simulink model "test_d_v_p"  (Simulink 6.2)
settings: Solver=ode45  StartTime=0.0  StopTime=30000  RelTol=1e-3
undefined symbols (not defined in the file or in its folder): ant_bits, blockCountBits, blockRowBits
libraries: xbsIndex_r3 x843, xps_library x50, casper_library x17
(part 1 of 6)
settings Model: LastModifiedBy=Jason Manley
settings DebuggingCC: SolverPrmCheckMsg=warning

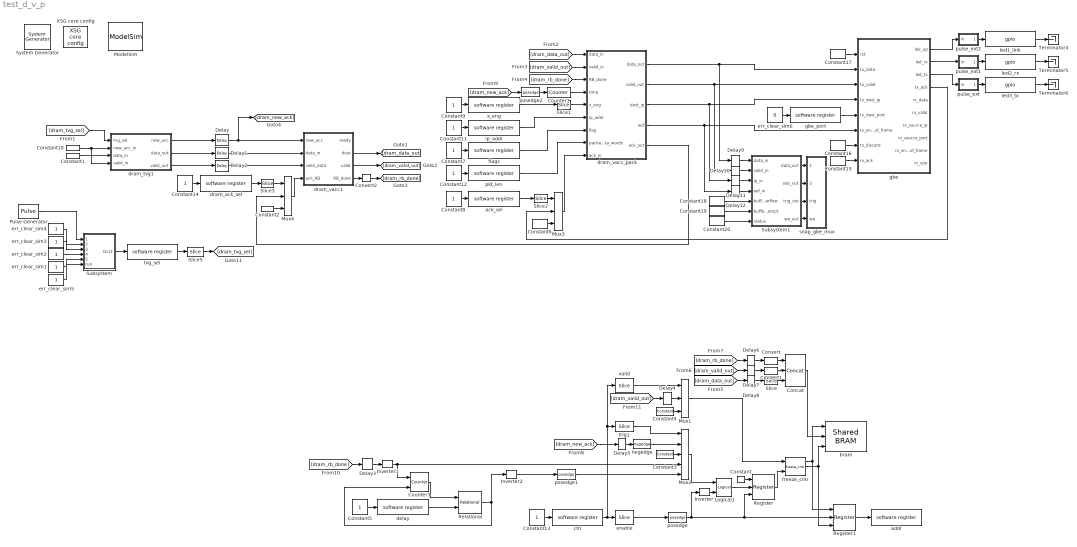
== system test_d_v_p ==
  " System Generator" : xbsIndex_r3/ System Generator  Tag=genX  xilinxfamily=Virtex2P  part=xc2vp70  speed=-7  package=ff1704  synthesis_tool=XST  directory=./test_d_v_p/sysgen  testbench=off  simulink_period=1  sysclk_period=4.878  incr_netlist=off  trim_vbits=Everywhere in SubSystem  dbl_ovrd=According to Block Masks  core_generation=According to Block Masks  run_coregen=off  deprecated_control=off  eval_field=0
      settings: AttributesFormatString=System\nGenerator
  Concat : xbsIndex_r3/Concat  num_inputs=3  explicit_period=off  period=1  dbl_ovrd=off
  Constant{,2..4} (4 alike) : xbsIndex_r3/Constant  const=1  equ=P=C  arith_type=Boolean  n_bits=1  bin_pt=0  opselect=C  inp2=PCIN>>17  opr=+  inp1=P  carry=CIN  iostate=0  explicit_period=on  period=1  dbl_ovrd=off
  Constant1 : xbsIndex_r3/Constant  const=0  equ=P=C  arith_type=Unsigned  n_bits=128  bin_pt=0  opselect=C  inp2=PCIN>>17  opr=+  inp1=P  carry=CIN  iostate=0  explicit_period=on  period=1  dbl_ovrd=off
  Constant10 : xbsIndex_r3/Constant  const=0  equ=P=C  arith_type=Boolean  n_bits=1  bin_pt=0  opselect=C  inp2=PCIN>>17  opr=+  inp1=P  carry=CIN  iostate=0  explicit_period=on  period=1  dbl_ovrd=off
  Constant{5,7..9,11..14} (8 alike) : Constant
  Constant15 : xbsIndex_r3/Constant  const=1  equ=P=C  arith_type=Boolean  n_bits=32  bin_pt=0  opselect=C  inp2=PCIN>>17  opr=+  inp1=P  carry=CIN  iostate=0  explicit_period=on  period=1  dbl_ovrd=off
  Constant{16..19} (4 alike) : xbsIndex_r3/Constant  const=0  equ=P=C  arith_type=Boolean  n_bits=32  bin_pt=0  opselect=C  inp2=PCIN>>17  opr=+  inp1=P  carry=CIN  iostate=0  explicit_period=on  period=1  dbl_ovrd=off
  Constant20 : xbsIndex_r3/Constant  const=0  equ=P=C  arith_type=Unsigned  n_bits=9  bin_pt=0  opselect=C  inp2=PCIN>>17  opr=+  inp1=P  carry=CIN  iostate=0  explicit_period=on  period=1  dbl_ovrd=off
  Constant6 : xbsIndex_r3/Constant  const=1  equ=P=C  arith_type=Boolean  n_bits=32  bin_pt=0  opselect=C  inp2=PCIN>>17  opr=+  inp1=P  carry=CIN  iostate=0  explicit_period=on  period=1  dbl_ovrd=off
  Convert : xbsIndex_r3/Convert  arith_type=Unsigned  n_bits=1  bin_pt=0  quantization=Truncate  overflow=Wrap  latency=0  explicit_period=off  period=1  dbl_ovrd=off  show_param=off  inserted_by_tool=off  pipeline=off
      settings: xl_area=[0, 0, 0, 0, 0, 0, 0]
  Convert1 : xbsIndex_r3/Convert  arith_type=Unsigned  n_bits=1  bin_pt=0  quantization=Truncate  overflow=Wrap  latency=0  explicit_period=off  period=1  dbl_ovrd=off  show_param=off  inserted_by_tool=off  pipeline=off
      settings: xl_area=[0, 0, 0, 0, 0, 0, 0]
  Convert2 : xbsIndex_r3/Convert  arith_type=Boolean  n_bits=1  bin_pt=0  quantization=Truncate  overflow=Wrap  latency=0  explicit_period=off  period=1  dbl_ovrd=off  show_param=off  inserted_by_tool=off  pipeline=off
      settings: xl_area=[0, 0, 0, 0, 0, 0, 0]
  Counter1 : xbsIndex_r3/Counter  cnt_type=Free Running  n_bits=64  bin_pt=0  arith_type=Unsigned  start_count=0  cnt_to=1023  cnt_by_val=1  operation=Up  explicit_period=on  period=1  load_pin=off  rst=off  en=on  dbl_ovrd=off  show_param=off  use_rpm=on  gen_core=off
      settings: xl_area=[0, 0, 0, 0, 0, 0, 0]
  Counter3 : xbsIndex_r3/Counter  cnt_type=Free Running  n_bits=32  bin_pt=0  arith_type=Unsigned  start_count=0  cnt_to=1023  cnt_by_val=1  operation=Up  explicit_period=on  period=1  load_pin=off  rst=on  en=on  dbl_ovrd=off  show_param=off  use_rpm=on  gen_core=off
      settings: xl_area=[0, 0, 0, 0, 0, 0, 0]
  Delay{,1..12} (13 alike) : xbsIndex_r3/Delay  latency=5  reg_retiming=on  explicit_period=off  period=1  en=off  accept_only_valid=off  init_zero=on  dbl_ovrd=off  show_param=off
      settings: xl_area=[0, 0, 0, 0, 0, 0, 0]
  Inverter : xbsIndex_r3/Inverter  latency=0  explicit_period=off  period=1  en=off  dbl_ovrd=off  show_param=off
      settings: xl_area=[0, 0, 0, 0, 0, 0, 0]
  Inverter1 : xbsIndex_r3/Inverter  latency=0  explicit_period=off  period=1  en=off  dbl_ovrd=off  show_param=off
      settings: xl_area=[0, 0, 0, 0, 0, 0, 0]
  Inverter2 : xbsIndex_r3/Inverter  latency=0  explicit_period=off  period=1  en=off  dbl_ovrd=off  show_param=off
      settings: xl_area=[0, 0, 0, 0, 0, 0, 0]
  Logical1 : xbsIndex_r3/Logical  logical_function=AND  inputs=2  precision=Full  arith_type=Unsigned  n_bits=8  bin_pt=2  align_bp=on  latency=0  explicit_period=off  period=1  en=off  dbl_ovrd=off  show_param=off
      settings: xl_area=[0, 0, 0, 0, 0, 0, 0]
  ModelSim : xbsIndex_r3/ModelSim  dir=./modelsim  waveform=on  leave_open=on  skip_compile=off  custom_scripts=off  startup_timeout=40
  Mux1 : xbsIndex_r3/Mux  inputs=2  precision=Full  arith_type="Signed  (2's comp)"  n_bits=8  bin_pt=2  quantization=Truncate  overflow=Wrap  latency=0  explicit_period=off  period=1  en=off  dbl_ovrd=off  show_param=off  mux_type=off  use_rpm=off  gen_core=off
      settings: xl_area=[0, 0, 0, 0, 0, 0, 0]
  Mux2 : xbsIndex_r3/Mux  inputs=4  precision=Full  arith_type="Signed  (2's comp)"  n_bits=8  bin_pt=2  quantization=Truncate  overflow=Wrap  latency=0  explicit_period=off  period=1  en=off  dbl_ovrd=off  show_param=off  mux_type=off  use_rpm=off  gen_core=off
      settings: xl_area=[0, 0, 0, 0, 0, 0, 0]
  Mux3 : xbsIndex_r3/Mux  inputs=2  precision=Full  arith_type="Signed  (2's comp)"  n_bits=8  bin_pt=2  quantization=Truncate  overflow=Wrap  latency=0  explicit_period=off  period=1  en=off  dbl_ovrd=off  show_param=off  mux_type=off  use_rpm=off  gen_core=off
      settings: xl_area=[0, 0, 0, 0, 0, 0, 0]
  Mux4 : xbsIndex_r3/Mux  inputs=2  precision=Full  arith_type="Signed  (2's comp)"  n_bits=8  bin_pt=2  quantization=Truncate  overflow=Wrap  latency=0  explicit_period=off  period=1  en=off  dbl_ovrd=off  show_param=off  mux_type=off  use_rpm=off  gen_core=off
      settings: xl_area=[0, 0, 0, 0, 0, 0, 0]
  Pulse Generator : DiscretePulseGenerator  Period=3000  PhaseDelay=600
  Register : xbsIndex_r3/Register  init=0  reg_only_valid=off  explicit_period=off  period=1  rst=on  en=on  out_en=off  dbl_ovrd=off  show_param=off
      settings: xl_area=[0, 0, 0, 0, 0, 0, 0]
  Register1 : xbsIndex_r3/Register  init=0  reg_only_valid=off  explicit_period=off  period=1  rst=on  en=on  out_en=off  dbl_ovrd=off  show_param=off
      settings: xl_area=[0, 0, 0, 0, 0, 0, 0]
  Relational : xbsIndex_r3/Relational  mode=a<=b  latency=0  explicit_period=off  period=1  en=off  dbl_ovrd=off  show_param=off
      settings: xl_area=[0, 0, 0, 0, 0, 0, 0]
  Slice : xbsIndex_r3/Slice  mode=Lower Bit Location + Width  nbits=30  bit1=0  base1=MSB of Input  bit0=0  base0=LSB of Input  boolean_output=off  explicit_period=off  period=1  dbl_ovrd=off
  Slice1 : xbsIndex_r3/Slice  mode=Lower Bit Location + Width  nbits=16  bit1=0  base1=MSB of Input  bit0=0  base0=LSB of Input  boolean_output=off  explicit_period=off  period=1  dbl_ovrd=off
  Slice2 : xbsIndex_r3/Slice  mode=Lower Bit Location + Width  nbits=1  bit1=0  base1=MSB of Input  bit0=0  base0=LSB of Input  boolean_output=off  explicit_period=off  period=1  dbl_ovrd=off
  Slice3 : xbsIndex_r3/Slice  mode=Lower Bit Location + Width  nbits=1  bit1=0  base1=MSB of Input  bit0=0  base0=LSB of Input  boolean_output=off  explicit_period=off  period=1  dbl_ovrd=off
  Slice5 : xbsIndex_r3/Slice  mode=Lower Bit Location + Width  nbits=6  bit1=0  base1=MSB of Input  bit0=9  base0=LSB of Input  boolean_output=off  explicit_period=off  period=1  dbl_ovrd=off
  Subsystem : Subsystem
  Subsystem1 : Subsystem
  Terminator4 : Terminator
  Terminator5 : Terminator
  Terminator6 : Terminator
  XSG core config : xps_library/XSG core config  Tag=xps:xsg  hw_sys=BEE2_usr  ibob_linux=off  clk_src=sys_clk2x  gpio_clk_io_group=iBOB:sma  gpio_clk_bit_index=0  clk_rate=205  sample_period=1  synthesis_tool=XST  mpc_type=powerpc405
  ack_sel : xps_library/software register  Tag=xps:sw_reg  io_dir=From Processor  arith_type=Unsigned  bitwidth=32  bin_pt=0  sample_period=1  gw_name=test_d_v_p_ack_sel_user_data_out
  addr : xps_library/software register  Tag=xps:sw_reg  io_dir=To Processor  arith_type=Unsigned  bitwidth=32  bin_pt=0  sample_period=1  gw_name=test_d_v_p_addr_user_data_in
  bram : xps_library/Shared BRAM  Tag=xps:bram  arith_type=Unsigned  addr_width=14  data_width=32  data_bin_pt=0  init_vals=0  sample_rate=1
  ctrl : xps_library/software register  Tag=xps:sw_reg  io_dir=From Processor  arith_type=Unsigned  bitwidth=32  bin_pt=0  sample_period=1  gw_name=test_d_v_p_ctrl_user_data_out
  delay : xps_library/software register  Tag=xps:sw_reg  io_dir=From Processor  arith_type=Unsigned  bitwidth=32  bin_pt=0  sample_period=1  gw_name=test_d_v_p_delay_user_data_out
  dram_ack_sel : xps_library/software register  Tag=xps:sw_reg  io_dir=From Processor  arith_type=Unsigned  bitwidth=32  bin_pt=0  sample_period=1  gw_name=test_d_v_p_dram_ack_sel_user_data_out
  dram_tvg1 : Subsystem  mask{len=100}
      mask prompts: len "Number of Vectors"
      mask init:
      | fmtstr = sprintf('Vector Length: %d', len);
      | set_param(gcb, 'AttributesFormatString', fmtstr);
      settings: AttributesFormatString=Vector Length: 100
  dram_vacc1 : Subsystem  mask{acc_length=100}
      mask prompts: acc_length "Vector length??(# cycles)"
      mask init:
      | valid_length = 36;
  dram_vacc_pack : Subsystem  mask{vector_len=100}
      mask prompts: vector_len "vector length"
  enable : xbsIndex_r3/Slice  mode=Lower Bit Location + Width  nbits=1  bit1=0  base1=LSB of Input  bit0=0  base0=LSB of Input  boolean_output=on  explicit_period=off  period=1  dbl_ovrd=off
  err_clear_sim{1..5} (5 alike) : Constant
  err_clear_sim6 : Constant  Value=0
  flags : xps_library/software register  Tag=xps:sw_reg  io_dir=From Processor  arith_type=Unsigned  bitwidth=32  bin_pt=0  sample_period=1  gw_name=test_d_v_p_flags_user_data_out
  freeze_cntr : casper_library/Misc/freeze_cntr  CounterBits=14
  gbe : Subsystem  Tag=xps:tengbe  AncestorBlock=xps_library/ten_GbE  mask{port=BEE2_usr:2, mac_lite=on, show_param=off, pre_emph=3, swing=800}
      mask prompts: mac_lite "Use light-weight MAC: Warning --> it DOES NOT check any CRC on receive"; show_param "---------------------- Show Implementation Parameters -----------------------------------------------------------------------------------"; pre_emph "Pre-emphasis"; swing "Differential swing"
      mask init:
      | tengbe_mask;
      mask StyleString: popup(iBOB:0|iBOB:1|BEE2_ctrl:0|BEE2_ctrl:1|BEE2_usr:0|BEE2_usr:1|BEE2_usr:2|BEE2_usr:3|CORR:0),checkbox,checkbox,popup(0|1|2|3),popup(400|500|600|700|800)
      mask CallbackString:
      | ||myname=gcb;
      | if strcmp(get_param(myname, 'show_param'), 'on')
      |     set_param(myname, 'MaskVisibilities', {'on','on','on','on', 'on'});
      | else
      |     set_param(myname, 'MaskVisibilities', {'on','on','on','off','off'});
      | end||
  gbe_port : xps_library/software register  Tag=xps:sw_reg  io_dir=From Processor  arith_type=Unsigned  bitwidth=32  bin_pt=0  sample_period=1  gw_name=test_d_v_p_gbe_port_user_data_out
  ip_addr : xps_library/software register  Tag=xps:sw_reg  io_dir=From Processor  arith_type=Unsigned  bitwidth=32  bin_pt=0  sample_period=1  gw_name=test_d_v_p_ip_addr_user_data_out
  led1_link : xps_library/gpio  Tag=xps:gpio  io_group=BEE2_usr:led  io_dir=out  arith_type=Boolean  bitwidth=1  bin_pt=0  bit_index=0  sample_period=1  use_single_ended=off  use_ddr=off  reg_iob=off  reg_clk_phase=0  termination=None
  led2_rx : xps_library/gpio  Tag=xps:gpio  io_group=BEE2_usr:led  io_dir=out  arith_type=Boolean  bitwidth=1  bin_pt=0  bit_index=1  sample_period=1  use_single_ended=off  use_ddr=off  reg_iob=off  reg_clk_phase=0  termination=None
  led3_tx : xps_library/gpio  Tag=xps:gpio  io_group=BEE2_usr:led  io_dir=out  arith_type=Boolean  bitwidth=1  bin_pt=0  bit_index=2  sample_period=1  use_single_ended=off  use_ddr=off  reg_iob=off  reg_clk_phase=0  termination=None
  negedge : casper_library/Misc/negedge  Tag=Rising Edge Detector
  pkt_len : xps_library/software register  Tag=xps:sw_reg  io_dir=From Processor  arith_type=Unsigned  bitwidth=32  bin_pt=0  sample_period=1  gw_name=test_d_v_p_pkt_len_user_data_out
  posedge : casper_library/Misc/posedge  Tag=Rising Edge Detector
  posedge1 : casper_library/Misc/posedge  Tag=Rising Edge Detector
  posedge2 : casper_library/Misc/posedge  Tag=Rising Edge Detector
  pulse_ext : Subsystem  mask{pulse_len=2^23}
      mask prompts: pulse_len "Length of Pulse"
      mask init:
      | bits = ceil(log2(pulse_len));
  pulse_ext1 : Subsystem  mask{pulse_len=2^23}
      mask prompts: pulse_len "Length of Pulse"
      mask init:
      | bits = ceil(log2(pulse_len));
  pulse_ext2 : Subsystem  mask{pulse_len=2^23}
      mask prompts: pulse_len "Length of Pulse"
      mask init:
      | bits = ceil(log2(pulse_len));
  snap_gbe_mux : Subsystem  AncestorBlock=casper_library/Scopes/snap64  mask(snap64){nsamples=11}
      mask prompts: nsamples "No. of samples(2^?)"
      mask help:
      | The <i>snap</i> block provides a packaged solution to capturing data from
      | the FPGA fabric and making it accessible from the CPU.  The block comes in
      | 2 flavors: <i>snap</i> (which captures to a 32 bit wide Shared BRAM), and
      | <i>snap64</i> (which captures to 2x32 bit wide Shared BRAMs to effect a
      | 64 bit capture).
      mask Help: eval('xlWeb([getenv(''MLIB_ROOT''), ''\casper_library\doc\snap_usage.html''])')
  trig1 : xbsIndex_r3/Slice  mode=Lower Bit Location + Width  nbits=2  bit1=0  base1=LSB of Input  bit0=1  base0=LSB of Input  boolean_output=on  explicit_period=off  period=1  dbl_ovrd=off
  tvg_sel : xps_library/software register  Tag=xps:sw_reg  io_dir=From Processor  arith_type=Unsigned  bitwidth=32  bin_pt=0  sample_period=1  gw_name=test_d_v_p_tvg_sel_user_data_out
  valid : xbsIndex_r3/Slice  mode=Lower Bit Location + Width  nbits=1  bit1=0  base1=LSB of Input  bit0=3  base0=LSB of Input  boolean_output=on  explicit_period=off  period=1  dbl_ovrd=off
  x_eng : xps_library/software register  Tag=xps:sw_reg  io_dir=From Processor  arith_type=Unsigned  bitwidth=32  bin_pt=0  sample_period=1  gw_name=test_d_v_p_x_eng_user_data_out
  wires:
  dram_vacc1/3(valid) -> [dram_valid_out]
  dram_vacc1/4(RB_done) -> Convert2/1
  tvg_sel/1 -> Slice5/1
  Slice5/1 -> [dram_tvg_sel]
  [dram_tvg_sel] -> dram_tvg1/1(tvg_sel)
  Constant10/1 -> dram_tvg1/4(valid_in), dram_tvg1/2(new_acc_in)
  Constant1/1 -> dram_tvg1/3(data_in)
  err_clear_sim1/1 -> Subsystem/5(data_sel)
  err_clear_sim2/1 -> Subsystem/4(valid_sel)
  err_clear_sim3/1 -> Subsystem/3(inj_vector)
  err_clear_sim4/1 -> Subsystem/2(inj_counter)
  Subsystem/1(Out1) -> tvg_sel/1
  Pulse Generator/1 -> Subsystem/1(new_acc)
  err_clear_sim5/1 -> Subsystem/6(run)
  dram_tvg1/1(new_acc) -> Delay/1
  dram_tvg1/2(data_out) -> Delay1/1
  dram_tvg1/3(valid_out) -> Delay2/1
  Convert/1 -> Concat/1
  Slice/1 -> Concat/3
  Convert1/1 -> Concat/2
  Mux2/1 -> Logical1/1
  Inverter/1 -> Logical1/2
  Logical1/1 -> Register/2
  valid/1 -> Mux1/1
  trig1/1 -> Mux2/1
  Register1/1 -> addr/1
  Constant4/1 -> Mux1/3
  Mux1/1 -> freeze_cntr/1
  Constant3/1 -> Mux2/3
  Constant/1 -> Register/1
  posedge/1 -> Inverter/1, Register1/2, Register/3
  ctrl/1 -> trig1/1, valid/1, enable/1
  Concat/1 -> bram/2
  Constant13/1 -> ctrl/1
  freeze_cntr/2 -> Register1/3, bram/3
  Register/1 -> freeze_cntr/2
  enable/1 -> posedge/1
  freeze_cntr/1 -> bram/1, Register1/1
  Inverter1/1 -> Mux2/4, Counter3/1
  negedge/1 -> Mux2/2
  Counter3/1 -> Relational/1
  delay/1 -> Relational/2
  Relational/1 -> Counter3/2, Inverter2/1
  Inverter2/1 -> posedge1/1
  posedge1/1 -> Mux2/5
  Constant5/1 -> delay/1
  Slice1/1 -> dram_vacc_pack/5(x_eng)
  pkt_len/1 -> dram_vacc_pack/8(packet_data_words)
  ip_addr/1 -> dram_vacc_pack/6(ip_addr)
  flags/1 -> dram_vacc_pack/7(flag)
  Constant12/1 -> pkt_len/1
  dram_vacc1/2(dout) -> [dram_data_out]
  [dram_data_out] -> dram_vacc_pack/1(data_in)
  [dram_valid_out] -> dram_vacc_pack/2(valid_in)
  [dram_rb_done] -> dram_vacc_pack/3(RB_done)
  Counter1/1 -> dram_vacc_pack/4(time)
  posedge2/1 -> Counter1/1
  x_eng/1 -> Slice1/1
  [dram_data_out] -> Delay8/1
  [dram_valid_out] -> Delay7/1
  [dram_rb_done] -> Delay6/1
  Constant9/1 -> x_eng/1
  Constant11/1 -> ip_addr/1
  Constant7/1 -> flags/1
  Mux3/1 -> dram_vacc_pack/9(ack_in)
  Constant6/1 -> Mux3/3
  gbe/4(tx_ack) -> Mux3/2
  pulse_ext/1(out) -> led3_tx/1
  pulse_ext1/1(out) -> led2_rx/1
  pulse_ext2/1(out) -> led1_link/1
  led1_link/1 -> Terminator4/1
  led2_rx/1 -> Terminator5/1
  led3_tx/1 -> Terminator6/1
  gbe/1(led_up) -> pulse_ext2/1(in)
  gbe/2(led_rx) -> pulse_ext1/1(in)
  gbe/3(led_tx) -> pulse_ext/1(in)
  Constant8/1 -> ack_sel/1
  Slice2/1 -> Mux3/1
  ack_sel/1 -> Slice2/1
  dram_vacc_pack/1(data_out) -> gbe/2(tx_data), Delay9/1
  dram_vacc_pack/2(valid_out) -> gbe/3(tx_valid), Delay10/1
  dram_vacc_pack/3(dest_ip) -> gbe/4(tx_dest_ip), Delay11/1
  dram_vacc_pack/4(eof) -> gbe/6(tx_end_of_frame), Delay12/1
  dram_vacc_pack/5(ack_out) -> Mux4/2
  [dram_new_ack] -> Delay5/1
  Mux4/1 -> dram_vacc1/4(ack_RB)
  Constant2/1 -> Mux4/3
  Constant14/1 -> dram_ack_sel/1
  Slice3/1 -> Mux4/1
  dram_ack_sel/1 -> Slice3/1
  Constant15/1 -> gbe/8(rx_ack)
  Constant16/1 -> gbe/7(tx_discard)
  err_clear_sim6/1 -> gbe_port/1
  gbe_port/1 -> gbe/5(tx_dest_port)
  Constant17/1 -> gbe/1(rst)
  [dram_new_ack] -> posedge2/1
  Subsystem1/1(data_out) -> snap_gbe_mux/1(data_in)
  Subsystem1/2(oob_out) -> snap_gbe_mux/2(oob_in)
  Subsystem1/3(trig_out) -> snap_gbe_mux/3(trig)
  Subsystem1/4(we_out) -> snap_gbe_mux/4(we)
  Constant18/1 -> Subsystem1/5(buffer_overflow)
  Constant19/1 -> Subsystem1/6(buffer_empt)
  Constant20/1 -> Subsystem1/7(status)
  Delay/1 -> [dram_new_ack], dram_vacc1/1(new_acc)
  Delay1/1 -> dram_vacc1/2(data_in)
  Delay2/1 -> dram_vacc1/3(valid_data)
  [dram_rb_done] -> Delay3/1
  [dram_valid_out] -> Delay4/1
  Delay3/1 -> Inverter1/1
  Delay4/1 -> Mux1/2
  Delay5/1 -> negedge/1
  Delay6/1 -> Convert/1
  Delay7/1 -> Convert1/1
  Delay8/1 -> Slice/1
  Delay9/1 -> Subsystem1/1(data_in)
  Delay10/1 -> Subsystem1/2(valid_in)
  Delay11/1 -> Subsystem1/3(ip_in)
  Delay12/1 -> Subsystem1/4(eof_in)
  Convert2/1 -> [dram_rb_done]

== system test_d_v_p/Subsystem ==
  new_acc : Inport  Port=1  LatchInput=off
  inj_counter : Inport  Port=2  LatchInput=off
  inj_vector : Inport  Port=3  LatchInput=off
  valid_sel : Inport  Port=4  LatchInput=off
  data_sel : Inport  Port=5  LatchInput=off
  run : Inport  Port=6  LatchInput=off
  Sum : Sum  Inputs=|++++++
  data_sel1 : Subsystem  mask{bit_pos=10}
      mask prompts: bit_pos "bit position"
  inj_counter1 : Subsystem  mask{bit_pos=13}
      mask prompts: bit_pos "bit position"
  inj_vector1 : Subsystem  mask{bit_pos=12}
      mask prompts: bit_pos "bit position"
  new_acc2 : Subsystem  mask{bit_pos=14}
      mask prompts: bit_pos "bit position"
  run1 : Subsystem  mask{bit_pos=9}
      mask prompts: bit_pos "bit position"
  valid_sel1 : Subsystem  mask{bit_pos=11}
      mask prompts: bit_pos "bit position"
  Out1 : Outport
  wires:
  new_acc2/1(Out1) -> Sum/1
  inj_counter1/1(Out1) -> Sum/2
  inj_vector1/1(Out1) -> Sum/3
  valid_sel1/1(Out1) -> Sum/4
  data_sel1/1(Out1) -> Sum/5
  run1/1(Out1) -> Sum/6
  new_acc/1 -> new_acc2/1(In1)
  inj_counter/1 -> inj_counter1/1(In1)
  inj_vector/1 -> inj_vector1/1(In1)
  valid_sel/1 -> valid_sel1/1(In1)
  Sum/1 -> Out1/1
  data_sel/1 -> data_sel1/1(In1)
  run/1 -> run1/1(In1)

== system test_d_v_p/Subsystem1 ==
  data_in : Inport  Port=1  LatchInput=off
  valid_in : Inport  Port=2  LatchInput=off
  ip_in : Inport  Port=3  LatchInput=off
  eof_in : Inport  Port=4  LatchInput=off
  buffer_overflow : Inport  Port=5  LatchInput=off
  buffer_empt : Inport  Port=6  LatchInput=off
  status : Inport  Port=7  LatchInput=off
  Concat1 : xbsIndex_r3/Concat  num_inputs=5  explicit_period=off  period=1  dbl_ovrd=off
  Delay{1,4..6} (4 alike) : xbsIndex_r3/Delay  latency=2  reg_retiming=on  explicit_period=off  period=1  en=off  accept_only_valid=off  init_zero=on  dbl_ovrd=off  show_param=off
      settings: xl_area=[0, 0, 0, 0, 0, 0, 0]
  Logical4 : xbsIndex_r3/Logical  logical_function=AND  inputs=2  precision=Full  arith_type=Unsigned  n_bits=8  bin_pt=2  align_bp=on  latency=0  explicit_period=on  period=1  en=off  dbl_ovrd=off  show_param=off
      settings: xl_area=[0, 0, 0, 0, 0, 0, 0]
  Slice11 : xbsIndex_r3/Slice  mode=Lower Bit Location + Width  nbits=32-9-1-1-1  bit1=0  base1=MSB of Input  bit0=0  base0=LSB of Input  boolean_output=on  explicit_period=off  period=1  dbl_ovrd=off
  data_out : Outport
  oob_out : Outport  Port=2
  trig_out : Outport  Port=3
  we_out : Outport  Port=4
  wires:
  Slice11/1 -> Concat1/1
  Concat1/1 -> Delay4/1
  data_in/1 -> Delay1/1
  ip_in/1 -> Slice11/1
  Delay1/1 -> data_out/1
  Delay4/1 -> oob_out/1
  Delay5/1 -> Logical4/2, we_out/1
  Logical4/1 -> trig_out/1
  Delay6/1 -> Logical4/1
  valid_in/1 -> Delay5/1
  eof_in/1 -> Concat1/2, Delay6/1
  buffer_overflow/1 -> Concat1/3
  buffer_empt/1 -> Concat1/4
  status/1 -> Concat1/5

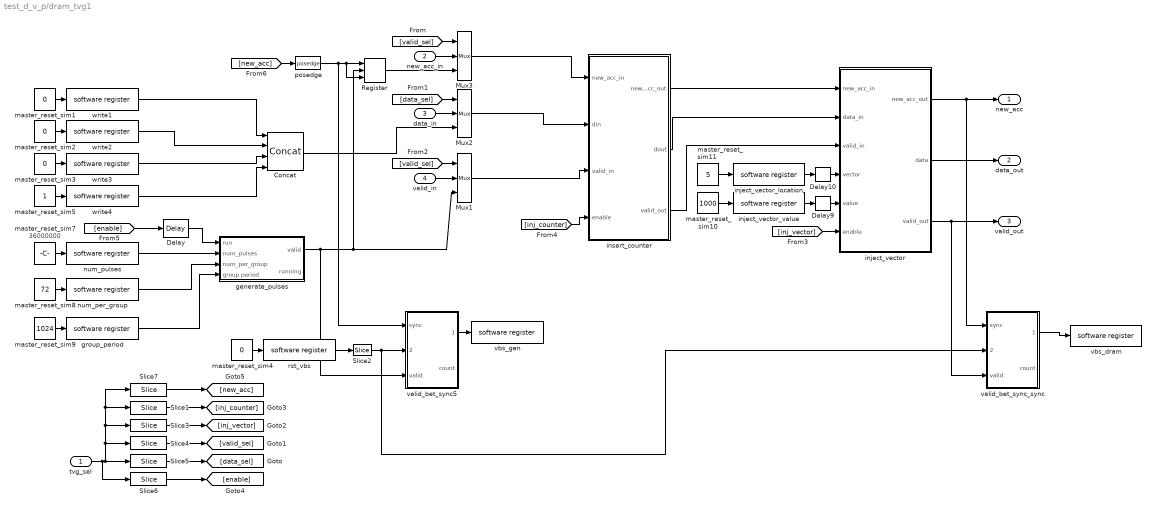
== system test_d_v_p/dram_tvg1 ==
  tvg_sel : Inport  Port=1  LatchInput=off
  new_acc_in : Inport  Port=2  LatchInput=off
  data_in : Inport  Port=3  LatchInput=off
  valid_in : Inport  Port=4  LatchInput=off
  Concat : xbsIndex_r3/Concat  num_inputs=4  explicit_period=on  period=1  dbl_ovrd=off
  Delay : xbsIndex_r3/Delay  latency=1  reg_retiming=on  explicit_period=off  period=1  en=off  accept_only_valid=off  init_zero=on  dbl_ovrd=off  show_param=off
      settings: xl_area=[0, 0, 0, 0, 0, 0, 0]
  Delay10 : xbsIndex_r3/Delay  latency=5  reg_retiming=off  explicit_period=off  period=1  en=off  accept_only_valid=off  init_zero=on  dbl_ovrd=off  show_param=off
      settings: xl_area=[0, 0, 0, 0, 0, 0, 0]
  Delay9 : xbsIndex_r3/Delay  latency=5  reg_retiming=off  explicit_period=off  period=1  en=off  accept_only_valid=off  init_zero=on  dbl_ovrd=off  show_param=off
      settings: xl_area=[0, 0, 0, 0, 0, 0, 0]
  Mux1 : xbsIndex_r3/Mux  inputs=2  precision=Full  arith_type="Signed  (2's comp)"  n_bits=8  bin_pt=2  quantization=Truncate  overflow=Wrap  latency=0  explicit_period=off  period=1  en=off  dbl_ovrd=off  show_param=off  mux_type=off  use_rpm=off  gen_core=off
      settings: xl_area=[0, 0, 0, 0, 0, 0, 0]
  Mux2 : xbsIndex_r3/Mux  inputs=2  precision=Full  arith_type="Signed  (2's comp)"  n_bits=8  bin_pt=2  quantization=Truncate  overflow=Wrap  latency=0  explicit_period=off  period=1  en=off  dbl_ovrd=off  show_param=off  mux_type=off  use_rpm=off  gen_core=off
      settings: xl_area=[0, 0, 0, 0, 0, 0, 0]
  Mux3 : xbsIndex_r3/Mux  inputs=2  precision=Full  arith_type="Signed  (2's comp)"  n_bits=8  bin_pt=2  quantization=Truncate  overflow=Wrap  latency=0  explicit_period=off  period=1  en=off  dbl_ovrd=off  show_param=off  mux_type=off  use_rpm=off  gen_core=off
      settings: xl_area=[0, 0, 0, 0, 0, 0, 0]
  Register : xbsIndex_r3/Register  init=0  reg_only_valid=off  explicit_period=off  period=1  rst=on  en=on  out_en=off  dbl_ovrd=off  show_param=off
      settings: xl_area=[0, 0, 0, 0, 0, 0, 0]
  Slice1 : xbsIndex_r3/Slice  mode=Lower Bit Location + Width  nbits=1  bit1=0  base1=MSB of Input  bit0=4  base0=LSB of Input  boolean_output=on  explicit_period=off  period=1  dbl_ovrd=off
  Slice2 : xbsIndex_r3/Slice  mode=Lower Bit Location + Width  nbits=1  bit1=0  base1=MSB of Input  bit0=0  base0=LSB of Input  boolean_output=on  explicit_period=off  period=1  dbl_ovrd=off
  Slice3 : xbsIndex_r3/Slice  mode=Lower Bit Location + Width  nbits=1  bit1=0  base1=MSB of Input  bit0=3  base0=LSB of Input  boolean_output=on  explicit_period=off  period=1  dbl_ovrd=off
  Slice4 : xbsIndex_r3/Slice  mode=Lower Bit Location + Width  nbits=1  bit1=0  base1=MSB of Input  bit0=2  base0=LSB of Input  boolean_output=on  explicit_period=off  period=1  dbl_ovrd=off
  Slice5 : xbsIndex_r3/Slice  mode=Lower Bit Location + Width  nbits=1  bit1=0  base1=MSB of Input  bit0=1  base0=LSB of Input  boolean_output=on  explicit_period=off  period=1  dbl_ovrd=off
  Slice6 : xbsIndex_r3/Slice  mode=Lower Bit Location + Width  nbits=1  bit1=0  base1=MSB of Input  bit0=0  base0=LSB of Input  boolean_output=on  explicit_period=off  period=1  dbl_ovrd=off
  Slice7 : xbsIndex_r3/Slice  mode=Lower Bit Location + Width  nbits=1  bit1=0  base1=MSB of Input  bit0=5  base0=LSB of Input  boolean_output=on  explicit_period=off  period=1  dbl_ovrd=off
  generate_pulses : Subsystem
  group_period : xps_library/software register  Tag=xps:sw_reg  io_dir=From Processor  arith_type=Unsigned  bitwidth=32  bin_pt=0  sample_period=1  gw_name=test_d_v_p_dram_tvg1_group_period_user_data_out
  inject_vector : Subsystem  mask{num_vectors=len}
      mask prompts: num_vectors "number of vectors"
      mask init:
      | fmtstr = sprintf('Vector Length: %d', num_vectors);
      | set_param(gcb, 'AttributesFormatString', fmtstr);
      settings: AttributesFormatString=Vector Length: 100
  inject_vector_location : xps_library/software register  Tag=xps:sw_reg  io_dir=From Processor  arith_type=Unsigned  bitwidth=32  bin_pt=0  sample_period=1  gw_name=test_d_v_p_dram_tvg1_inject_vector_location_user_data_out
  inject_vector_value : xps_library/software register  Tag=xps:sw_reg  io_dir=From Processor  arith_type=Unsigned  bitwidth=32  bin_pt=0  sample_period=1  gw_name=test_d_v_p_dram_tvg1_inject_vector_value_user_data_out
  insert_counter : Subsystem  mask{vec_len=len}
      mask prompts: vec_len "Vector Length?"
      mask init:
      | fmtstr = sprintf('Vector Length: %d', vec_len);
      | set_param(gcb, 'AttributesFormatString', fmtstr);
      settings: AttributesFormatString=Vector Length: 100
  master_reset_sim{1..4} (4 alike) : Constant  Value=0
  master_reset_sim10 : Constant  Value=1000
  master_reset_sim11 : Constant  Value=5
  master_reset_sim5 : Constant
  master_reset_sim7 : Constant  Value=36000000
  master_reset_sim8 : Constant  Value=72
  master_reset_sim9 : Constant  Value=1024
  num_per_group : xps_library/software register  Tag=xps:sw_reg  io_dir=From Processor  arith_type=Unsigned  bitwidth=32  bin_pt=0  sample_period=1  gw_name=test_d_v_p_dram_tvg1_num_per_group_user_data_out
  num_pulses : xps_library/software register  Tag=xps:sw_reg  io_dir=From Processor  arith_type=Unsigned  bitwidth=32  bin_pt=0  sample_period=1  gw_name=test_d_v_p_dram_tvg1_num_pulses_user_data_out
  posedge : casper_library/Misc/posedge  Tag=Rising Edge Detector
  rst_vbs : xps_library/software register  Tag=xps:sw_reg  io_dir=From Processor  arith_type=Unsigned  bitwidth=32  bin_pt=0  sample_period=1  gw_name=test_d_v_p_dram_tvg1_rst_vbs_user_data_out
  valid_bet_sync5 : Subsystem
  valid_bet_sync_sync : Subsystem
  vbs_dram : xps_library/software register  Tag=xps:sw_reg  io_dir=To Processor  arith_type=Unsigned  bitwidth=32  bin_pt=0  sample_period=1  gw_name=test_d_v_p_dram_tvg1_vbs_dram_user_data_in
  vbs_gen : xps_library/software register  Tag=xps:sw_reg  io_dir=To Processor  arith_type=Unsigned  bitwidth=32  bin_pt=0  sample_period=1  gw_name=test_d_v_p_dram_tvg1_vbs_gen_user_data_in
  write1 : xps_library/software register  Tag=xps:sw_reg  io_dir=From Processor  arith_type=Unsigned  bitwidth=32  bin_pt=0  sample_period=1  gw_name=test_d_v_p_dram_tvg1_write1_user_data_out
  write2 : xps_library/software register  Tag=xps:sw_reg  io_dir=From Processor  arith_type=Unsigned  bitwidth=32  bin_pt=0  sample_period=1  gw_name=test_d_v_p_dram_tvg1_write2_user_data_out
  write3 : xps_library/software register  Tag=xps:sw_reg  io_dir=From Processor  arith_type=Unsigned  bitwidth=32  bin_pt=0  sample_period=1  gw_name=test_d_v_p_dram_tvg1_write3_user_data_out
  write4 : xps_library/software register  Tag=xps:sw_reg  io_dir=From Processor  arith_type=Unsigned  bitwidth=32  bin_pt=0  sample_period=1  gw_name=test_d_v_p_dram_tvg1_write4_user_data_out
  new_acc : Outport
  data_out : Outport  Port=2
  valid_out : Outport  Port=3
  wires:
  write1/1 -> Concat/1
  master_reset_sim1/1 -> write1/1
  write2/1 -> Concat/2
  master_reset_sim2/1 -> write2/1
  write3/1 -> Concat/3
  master_reset_sim3/1 -> write3/1
  write4/1 -> Concat/4
  master_reset_sim5/1 -> write4/1
  [new_acc] -> posedge/1
  num_pulses/1 -> generate_pulses/2(num_pulses)
  master_reset_sim7/1 -> num_pulses/1
  num_per_group/1 -> generate_pulses/3(num_per_group)
  master_reset_sim8/1 -> num_per_group/1
  group_period/1 -> generate_pulses/4(group period)
  master_reset_sim9/1 -> group_period/1
  Mux1/1 -> insert_counter/3(valid_in)
  valid_in/1 -> Mux1/2
  inject_vector/1(new_acc_out) -> new_acc/1, valid_bet_sync_sync/1(sync)
  inject_vector/2(data) -> data_out/1
  inject_vector/3(valid_out) -> valid_out/1, valid_bet_sync_sync/3(valid)
  insert_counter/1(new_acc_out) -> inject_vector/1(new_acc_in)
  Mux2/1 -> insert_counter/2(din)
  data_in/1 -> Mux2/2
  new_acc_in/1 -> Mux3/2
  Mux3/1 -> insert_counter/1(new_acc_in)
  Slice5/1 -> [data_sel]
  tvg_sel/1 -> Slice5/1, Slice3/1, Slice1/1, Slice7/1, Slice4/1, Slice6/1
  Slice4/1 -> [valid_sel]
  [valid_sel] -> Mux3/1
  [data_sel] -> Mux2/1
  [valid_sel] -> Mux1/1
  Slice3/1 -> [inj_vector]
  Slice1/1 -> [inj_counter]
  [enable] -> Delay/1
  insert_counter/2(dout) -> inject_vector/2(data_in)
  insert_counter/3(valid_out) -> inject_vector/3(valid_in)
  Concat/1 -> Mux2/3
  generate_pulses/1(valid) -> Register/2, Mux1/3, valid_bet_sync5/3(valid)
  Register/1 -> Mux3/3
  posedge/1 -> Register/1, Register/3, valid_bet_sync5/1(sync)
  [inj_vector] -> inject_vector/6(enable)
  Delay10/1 -> inject_vector/4(vector)
  master_reset_sim11/1 -> inject_vector_location/1
  inject_vector_location/1 -> Delay10/1
  Delay9/1 -> inject_vector/5(value)
  master_reset_sim10/1 -> inject_vector_value/1
  inject_vector_value/1 -> Delay9/1
  [inj_counter] -> insert_counter/4(enable)
  Slice6/1 -> [enable]
  Slice7/1 -> [new_acc]
  valid_bet_sync5/1(max_count) -> vbs_gen/1
  master_reset_sim4/1 -> rst_vbs/1
  Slice2/1 -> valid_bet_sync5/2(rst_max), valid_bet_sync_sync/2(rst_max)
  rst_vbs/1 -> Slice2/1
  valid_bet_sync_sync/1(max_count) -> vbs_dram/1
  Delay/1 -> generate_pulses/1(run)
